simulink model "live_model"  (R2023b)
settings: Solver=VariableStepAuto  StartTime=0.0  StopTime=0.3  RelTol=1e-3
values from neighbouring files (symbols this model uses):
  Resistance_time_step = 0.2    [init_controller.m]
  RL_sim_final = 50    [init_controller.m]
  RL_sim_initial = 90    [init_controller.m]
  Ts = Tsw/50    (= 2.5e-07)    [init_controller.m]
  Tsc = 1/5000    (= 0.0002)    [init_controller.m]
  V0_sim = 130    [init_controller.m]
undefined symbols (not defined in the file or in its folder): DiscIntNeverNeededParam
libraries: fl_lib x7, nesl_utility x6, ee_lib x1, eePwmGenerator x1, simulink x1
settings Model: Creator=maxim  LastModifiedBy=maxim
settings OptimizationCC: ReuseModelBlockBuffer=off

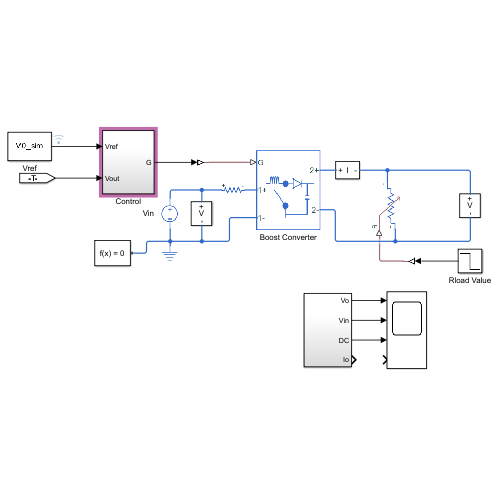
[thumbnail: Simulink's stored preview of the top-level diagram]
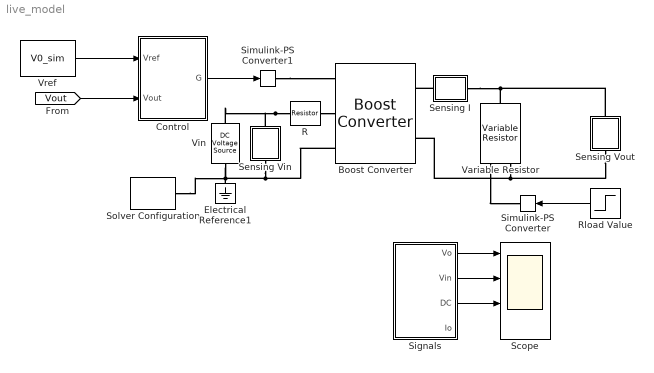
== system live_model ==
  Boost Converter : ee_lib/Semiconductors & Converters/Converters/Boost Converter  port_option=ee.enum.controlport.ps  device_type=4  Vf=0.8 V  Ron=1e-9 Ohm  Rds=0.01 Ohm  Goff=1e-6 1/Ohm  Vgt=1 V  Vgt_off=-1 V  Ih=1 A  Vth=0.5 V  K=0  diode_param=2  diode_Vf=0.8 V  diode_Ron=0.001 Ohm  diode_Goff=1e-5 1/Ohm  diode_C=50 nF  diode_iRM=-235 A  diode_iF=300 A  diode_idot=-50 A/us  diode_trr_param=1  diode_trr_factor=3  diode_trr=15 us  diode_Qrr=1500 s*uA  Lf=L.NominalValue H  Rl=18e-3 Ohm  Cf=Cap.NominalValue F  Rf=5e-3 Ohm  snubber_type=1  Cs=1e-7 F  Rs=0.1 Ohm  iL_specify=off  iL_priority=High  iL=0 A  iL_nominal_specify=off  iL_nominal_unit=A  iL_nominal_value=1  vc_specify=off  vc_priority=High  vc=0 V  vc_nominal_specify=off  vc_nominal_unit=V  vc_nominal_value=1
      settings: InternalSimscapePortConfiguration="{\"Bottom\":[],\"Left\":[{\"id\":\"G\",\"label\":\"G\",\"type\":\"input\"},{\"id\":\"p1\",\"label\":\"1+\",\"type\":\"foundation.electrical.electrical\"},{\"id\":\"n1\",\"label\":\"1-\",\"type\":\"foundation.electrical.electrical\"}],\"Right\":[{\"id\":\"p2\",\"label\":\"2+\",\"type\":\"foundation.electrical.electrical\"},{\"id\":\"n2\",\"label\":\"2-\",\"type\":\"foundation.electrical.electrical\"}],\"Top\":[]}"
  Control : Subsystem
  Electrical Reference1 : fl_lib/Electrical/Electrical Elements/Electrical Reference
  R : fl_lib/Electrical/Electrical Elements/Resistor  R=0.07 Ohm  i_specify=off  i_priority=None  i=0 A  i_nominal_specify=off  i_nominal_unit=A  i_nominal_value=1  v_specify=off  v_priority=None  v=0 V  v_nominal_specify=off  v_nominal_unit=V  v_nominal_value=1
  Rload Value : Step  Time=Resistance_time_step  Before=RL_sim_initial  After=RL_sim_final  SampleTime=0
  Scope : Scope  NumInputPorts=4
  Sensing Vin : Subsystem
      mask Display:
      | disp('V')
      | port_label('Lconn',1,'+')
      | port_label('Rconn',1,'-')
  Sensing Vout : Subsystem
      mask Display:
      | disp('V')
      | port_label('Lconn',1,'+')
      | port_label('Rconn',1,'-')
  Sensing I : Subsystem
      mask Display:
      | disp('I')
      | port_label('Lconn',1,'+')
      | port_label('Rconn',1,'-')
  Signals : Subsystem
  Simulink-PS Converter : nesl_utility/Simulink-PS Converter  PhysicalDomain=network_engine_domain  SubClassName=ps_input  LeftPortType=input  RightPortType=output  PseudoPeriodic=off  Frequencies=[]  NoiseDistribution=none  NoiseParameters=[]  Unit=1  AffineConversion=off  FilteringAndDerivatives=zero  SimscapeFilterOrder=1  InputFilterTimeConstant=0.001  UdotUserProvided=0
  Simulink-PS Converter1 : nesl_utility/Simulink-PS Converter  PhysicalDomain=network_engine_domain  SubClassName=ps_input  LeftPortType=input  RightPortType=output  PseudoPeriodic=off  Frequencies=[]  NoiseDistribution=none  NoiseParameters=[]  Unit=1  AffineConversion=off  FilteringAndDerivatives=provide  SimscapeFilterOrder=1  InputFilterTimeConstant=0.001  UdotUserProvided=0
  Solver Configuration : nesl_utility/Solver Configuration  PhysicalDomain=network_engine_domain  SubClassName=solver  LeftPortType=input  RightPortType=generic  Tones=[]  Harmonics=[]  SimulateNoise=off  Profile=off  UseLocalSampling=off  EnableSwitchedLinearOptims=on  FrequencyDomain=off  UseCCode=off  RelTol=0.001  AbsTol=1e-06  MinStep=1e-09  ToWorkspace=off  RevertToSquareIcSolve=off  NumHomotopyIterations=100  PhasorMode=off  PhasorModeNumHarmonics=1  ConsistencySolver=NEWTON_FTOL  IndexReductionMethod=DerivativeReplacement  DoDC=off  ResidualTolerance=1e-9  ConsistencyTolSource=GLOBAL  ConsistencyAbsTol=0.001  ConsistencyRelTol=0.001  ConsistencyTolFactor=0.001  UseLocalSolver=on  LocalSolverChoice=NE_BACKWARD_EULER_ADVANCER  ResolveIndetEquations=on  FunctionEvalNumThread=1  LocalSolverSampleTime=Ts  DoFixedCost=on  MaxNonlinIter=3  MaxModeIter=2  ComputeImpulses=off  ImpulseIterations=2  LinearAlgebra=auto  LinearAlgebraNumThread=0  EquationFormulation=NE_TIME_EF  DelaysMemoryBudget=1024  AutomaticFiltering=on  FilteringTimeConstant=0.001  PartitionStorageMethod=AS_NEEDED  PartitionMemoryBudget=1024  PartitionMethod=FAST  MultibodyUseLocalSolver=off  MultibodyLocalSolverChoice=ODE1  MultibodyLocalSolverSampleTime=0.001
  Variable Resistor : fl_lib/Electrical/Electrical Elements/Variable Resistor  Rmin=0 Ohm  thermalEnable=false  thermal_mass=1 J/K  i_specify=off  i_priority=None  i=0 A  i_nominal_specify=off  i_nominal_unit=A  i_nominal_value=1  v_specify=off  v_priority=None  v=0 V  v_nominal_specify=off  v_nominal_unit=V  v_nominal_value=1  T_specify=off  T_priority=None  T=300 K  T_nominal_specify=off  T_nominal_unit=K  T_nominal_value=1
  Vin : fl_lib/Electrical/Electrical Sources/DC Voltage Source  v0=Vi_sim_initial V
  Vref : Constant  Value=V0_sim  SampleTime=Ts
  wires:
  Signals/3(DC) -> Scope/3
  Control/1(G) -> Simulink-PS Converter1/1
  Rload Value/1 -> Simulink-PS Converter/1
  Vref/1 -> Control/1(Vref)
  Signals/2(Vin) -> Scope/2
  Signals/1(Vo) -> Scope/1
  [Vout] -> Control/2(Vout)
  connections:
  Sensing I/RConn1 -- Variable Resistor/RConn1 -- Sensing Vout/LConn1
  Sensing Vout/RConn1 -- Variable Resistor/LConn2 -- Boost Converter/RConn2
  Boost Converter/LConn3 -- Electrical Reference1/LConn1 -- Solver Configuration/RConn1 -- Vin/RConn1 -- Sensing Vin/RConn1
  R/LConn1 -- Vin/LConn1 -- Sensing Vin/LConn1
  R/RConn1 -- Boost Converter/LConn2
  Simulink-PS Converter1/RConn1 -- Boost Converter/LConn1
  Sensing I/LConn1 -- Boost Converter/RConn1
  Variable Resistor/LConn1 -- Simulink-PS Converter/RConn1

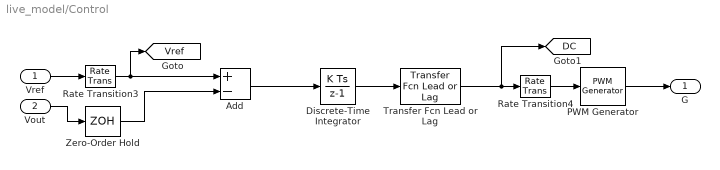
== system live_model/Control ==
  Vref : Inport
  Vout : Inport  Port=2
  Add : Sum  Inputs=+-
  Discrete-Time Integrator : DiscreteIntegrator  gainval=0.0010141  SampleTime=-1  ICPrevOutput=DiscIntNeverNeededParam  ICPrevScaledInput=DiscIntNeverNeededParam
  PWM Generator : eePwmGenerator/PWM Generator  CarrCount=Up  Tper=Tsw  Tdelay=0  Ts=Ts
  Rate Transition3 : RateTransition  OutPortSampleTime=Tsc
  Rate Transition4 : RateTransition  OutPortSampleTime=Ts
  Transfer Fcn Lead or Lag : simulink/Discrete/Transfer Fcn Lead or Lag  PoleZ=0.6672  ZeroZ=0.8742  ICPrevOutput=0.0  ICPrevInput=0.0  DoSatur=off
  Zero-Order Hold : ZeroOrderHold  SampleTime=Tsc
  G : Outport  VectorParamsAs1DForOutWhenUnconnected=off
  tag scope: DC=global, Vref=global
  wires:
  Vref/1 -> Rate Transition3/1
  Rate Transition3/1 -> Add/1, [Vref]
  Vout/1 -> Zero-Order Hold/1
  PWM Generator/1 -> G/1
  Transfer Fcn Lead or Lag/1 -> [DC], Rate Transition4/1
  Rate Transition4/1 -> PWM Generator/1
  Zero-Order Hold/1 -> Add/2
  Add/1 -> Discrete-Time Integrator/1
  Discrete-Time Integrator/1 -> Transfer Fcn Lead or Lag/1

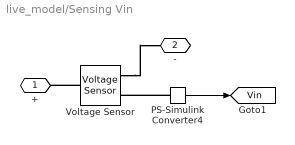
== system live_model/Sensing Vin ==
  PS-Simulink Converter4 : nesl_utility/PS-Simulink Converter  PhysicalDomain=network_engine_domain  SubClassName=ps_output  LeftPortType=input  RightPortType=output  PseudoPeriodic=off  Frequencies=[]  VectorFormat=1-D array  Unit=V  AffineConversion=off
  Voltage Sensor : fl_lib/Electrical/Electrical Sensors/Voltage Sensor
  + : PMIOPort  Side=Left
  - : PMIOPort  Port=2  Side=Right
  tag scope: Vin=global
  wires:
  PS-Simulink Converter4/1 -> [Vin]
  connections:
  Voltage Sensor/LConn1 -- +/RConn1
  Voltage Sensor/RConn2 -- -/RConn1
  PS-Simulink Converter4/LConn1 -- Voltage Sensor/RConn1

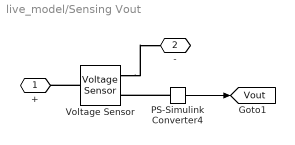
== system live_model/Sensing Vout ==
  PS-Simulink Converter4 : nesl_utility/PS-Simulink Converter  PhysicalDomain=network_engine_domain  SubClassName=ps_output  LeftPortType=input  RightPortType=output  PseudoPeriodic=off  Frequencies=[]  VectorFormat=1-D array  Unit=V  AffineConversion=off
  Voltage Sensor : fl_lib/Electrical/Electrical Sensors/Voltage Sensor
  + : PMIOPort  Side=Left
  - : PMIOPort  Port=2  Side=Right
  tag scope: Vout=global
  wires:
  PS-Simulink Converter4/1 -> [Vout]
  connections:
  Voltage Sensor/LConn1 -- +/RConn1
  Voltage Sensor/RConn2 -- -/RConn1
  PS-Simulink Converter4/LConn1 -- Voltage Sensor/RConn1

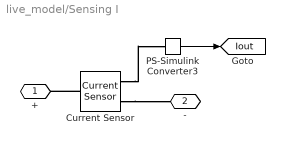
== system live_model/Sensing I ==
  Current Sensor : fl_lib/Electrical/Electrical Sensors/Current Sensor
  PS-Simulink Converter3 : nesl_utility/PS-Simulink Converter  PhysicalDomain=network_engine_domain  SubClassName=ps_output  LeftPortType=input  RightPortType=output  PseudoPeriodic=off  Frequencies=[]  VectorFormat=1-D array  Unit=A  AffineConversion=off
  + : PMIOPort  Side=Left
  - : PMIOPort  Port=2  Side=Right
  tag scope: Iout=global
  wires:
  PS-Simulink Converter3/1 -> [Iout]
  connections:
  Current Sensor/RConn2 -- -/RConn1
  Current Sensor/LConn1 -- +/RConn1
  Current Sensor/RConn1 -- PS-Simulink Converter3/LConn1

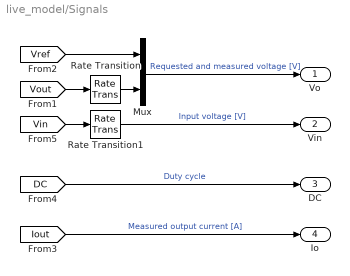
== system live_model/Signals ==
  Mux : Mux  Inputs=2
  Rate Transition : RateTransition  OutPortSampleTime=Tsc
  Rate Transition1 : RateTransition  OutPortSampleTime=Tsc
  Vo : Outport  VectorParamsAs1DForOutWhenUnconnected=off
  Vin : Outport  Port=2  VectorParamsAs1DForOutWhenUnconnected=off
  DC : Outport  Port=3  VectorParamsAs1DForOutWhenUnconnected=off
  Io : Outport  Port=4  VectorParamsAs1DForOutWhenUnconnected=off
  wires:
  [Vout] -> Rate Transition/1
  [Vin] -> Rate Transition1/1
  Rate Transition1/1 -> Vin/1  "Input voltage [V]"
  Mux/1 -> Vo/1  "Requested and measured voltage [V]"
  [Iout] -> Io/1  "Measured output current [A]"
  [Vref] -> Mux/1
  Rate Transition/1 -> Mux/2
  [DC] -> DC/1  "Duty cycle"
